simulink model "MotorAsincronoMotorCCCarga"  (Simulink 6.5)
settings: Solver=ode23t  StartTime=0.0  StopTime=4.5  RelTol=1e-6
undefined symbols (not defined in the file): powergui
libraries: powerlib x30, powerlib_extras x3
settings Model: Creator=RS  LastModifiedBy=PC_0
settings SolverCC: SolverResetMethod=Robust

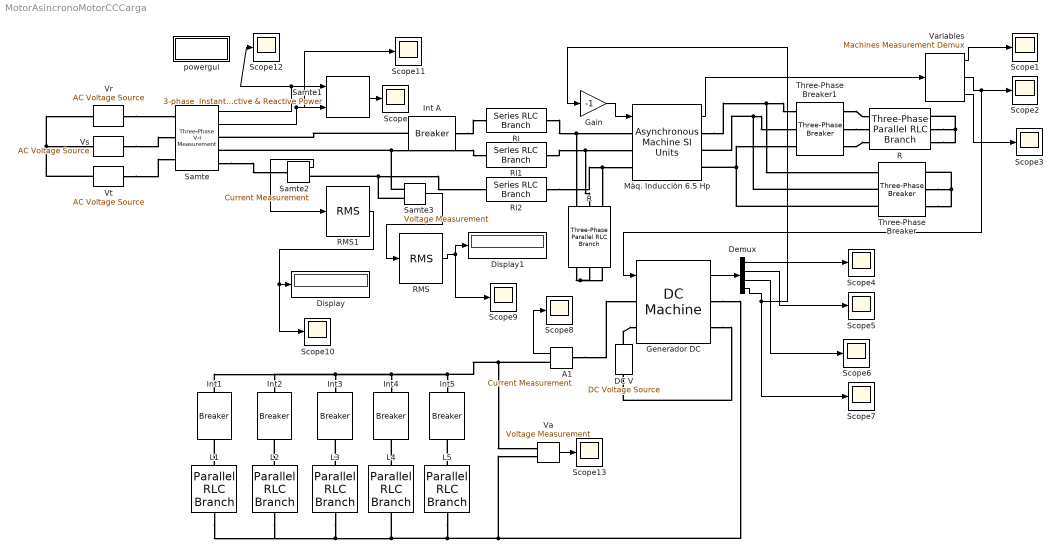
== system MotorAsincronoMotorCCCarga ==
  A1 : powerlib/Measurements/Current Measurement  Orientation=left  DialogController=PMDialogs.PMDefaultMaskDlg  SystemSampleTime=-1  PhasorSimulation=off  OutputType=Complex  PSBequivalent=0
  DC V : powerlib/Electrical Sources/DC Voltage Source  Orientation=up  DialogController=PMDialogs.PMDefaultMaskDlg  SystemSampleTime=-1  Amplitude=190  Measurements=None
  Demux : Demux
  Display : Display
  Display1 : Display
  Gain : Gain  Gain=-1
  Generador DC : powerlib/Machines/DC Machine  DialogController=PMDialogs.PMDefaultMaskDlg  SystemSampleTime=-1  PresetModel=No  MechanicalLoad=Speed w  ShowDetailedParameters=on  RLa="[ 0.5  0.01]"  RLf="[ 240  120]"  Laf=1.8  J=0.05  Bm=0.02  Tf=0  w0=0
  Int A : powerlib/Elements/Breaker  DialogController=PMDialogs.PMDefaultMaskDlg  SystemSampleTime=-1  BreakerResistance=0.01  InitialState=1  SnubberResistance=1e6  SnubberCapacitance=inf  SwitchingTimes=9  External=off  Measurements=None  MoreParameters=off  NoBreakLoop=off
  Int1 : powerlib/Elements/Breaker  Orientation=down  DialogController=PMDialogs.PMDefaultMaskDlg  SystemSampleTime=-1  BreakerResistance=0.01  InitialState=0  SnubberResistance=1e6  SnubberCapacitance=inf  SwitchingTimes=1.5  External=off  Measurements=None  MoreParameters=off  NoBreakLoop=off
  Int2 : powerlib/Elements/Breaker  Orientation=down  DialogController=PMDialogs.PMDefaultMaskDlg  SystemSampleTime=-1  BreakerResistance=0.01  InitialState=0  SnubberResistance=1e6  SnubberCapacitance=inf  SwitchingTimes=1.75  External=off  Measurements=None  MoreParameters=off  NoBreakLoop=off
  Int3 : powerlib/Elements/Breaker  Orientation=down  DialogController=PMDialogs.PMDefaultMaskDlg  SystemSampleTime=-1  BreakerResistance=0.01  InitialState=0  SnubberResistance=1e6  SnubberCapacitance=inf  SwitchingTimes=2  External=off  Measurements=None  MoreParameters=off  NoBreakLoop=off
  Int4 : powerlib/Elements/Breaker  Orientation=down  DialogController=PMDialogs.PMDefaultMaskDlg  SystemSampleTime=-1  BreakerResistance=0.01  InitialState=0  SnubberResistance=1e6  SnubberCapacitance=inf  SwitchingTimes=2.25  External=off  Measurements=None  MoreParameters=off  NoBreakLoop=off
  Int5 : powerlib/Elements/Breaker  Orientation=down  DialogController=PMDialogs.PMDefaultMaskDlg  SystemSampleTime=-1  BreakerResistance=0.01  InitialState=0  SnubberResistance=1e6  SnubberCapacitance=inf  SwitchingTimes=2.5  External=off  Measurements=None  MoreParameters=off  NoBreakLoop=off
  L{1..5} (5 alike) : powerlib/Elements/Parallel RLC Branch  Orientation=down  DialogController=PMDialogs.PMDefaultMaskDlg  PhysicalDomain=powersysdomain  SubClassName=unknown  LeftPortType=p1  RightPortType=p1  LConnTagsString=a  RConnTagsString=__new0  BranchType=R  Resistance=65  Inductance=1e-3  SetiL0=off  InitialCurrent=0  Capacitance=1e-6  Setx0=off  InitialVoltage=0  Measurements=None
  Màq. Inducciòn 6.5 Hp : powerlib/Machines/Asynchronous Machine SI Units  DialogController=PMDialogs.PMDefaultMaskDlg  SystemSampleTime=-1  PresetModel=No  MechanicalLoad=Torque Tm  ShowDetailedParameters=on  RotorType=Wound  ReferenceFrame=Stationary  NominalParameters="[6.5*746    380   50]"  Stator="[0.03   0.00006]"  Rotor="[1.094  0.00496]"  Lm=0.105  Mechanical="[0.041    0.001   2]"  PolePairs=2  InitialConditions="[ 1,0   0,0,0   0,0,0 ]"  Units=1  LoadFlowParameters=0  SimulateSaturation=on  Saturation=[ 0.5 3,6,9,12,15,18,30,50;20,190,380,400,420,440,450,451,452]
  R : powerlib/Elements/Three-Phase Parallel RLC Branch  DialogController=PMDialogs.PMDefaultMaskDlg  PhysicalDomain=powersysdomain  SubClassName=unknown  LeftPortType=p1  RightPortType=p1  LConnTagsString=A|B|C  RConnTagsString=A|B|C  BranchType=R  Resistance=4.2  Inductance=1e-3  Capacitance=1e-6  Measurements=None
  "R " : powerlib/Elements/Three-Phase Parallel RLC Branch  Orientation=down  DialogController=PMDialogs.PMDefaultMaskDlg  PhysicalDomain=powersysdomain  SubClassName=unknown  LeftPortType=p1  RightPortType=p1  LConnTagsString=A|B|C  RConnTagsString=A|B|C  BranchType=R  Resistance=300  Inductance=1e-3  Capacitance=1e-6  Measurements=None
  RMS : powerlib_extras/Measurements/RMS  DialogController=PMDialogs.PMDefaultMaskDlg  SystemSampleTime=-1  f1=50
  RMS1 : powerlib_extras/Measurements/RMS  DialogController=PMDialogs.PMDefaultMaskDlg  SystemSampleTime=-1  f1=50
  Rl : powerlib/Elements/Series RLC Branch  DialogController=PMDialogs.PMDefaultMaskDlg  PhysicalDomain=powersysdomain  SubClassName=unknown  LeftPortType=p1  RightPortType=p1  LConnTagsString=__new0  RConnTagsString=__new0  BranchType=RL  Resistance=0.6  Inductance=0.0049  SetiL0=off  InitialCurrent=0  Capacitance=1e-6  Setx0=off  InitialVoltage=0  Measurements=None
  Rl1 : powerlib/Elements/Series RLC Branch  DialogController=PMDialogs.PMDefaultMaskDlg  PhysicalDomain=powersysdomain  SubClassName=unknown  LeftPortType=p1  RightPortType=p1  LConnTagsString=__new0  RConnTagsString=__new0  BranchType=RL  Resistance=0.6  Inductance=0.0049  SetiL0=off  InitialCurrent=0  Capacitance=1e-6  Setx0=off  InitialVoltage=0  Measurements=None
  Rl2 : powerlib/Elements/Series RLC Branch  DialogController=PMDialogs.PMDefaultMaskDlg  PhysicalDomain=powersysdomain  SubClassName=unknown  LeftPortType=p1  RightPortType=p1  LConnTagsString=__new0  RConnTagsString=__new0  BranchType=RL  Resistance=0.6  Inductance=0.0049  SetiL0=off  InitialCurrent=0  Capacitance=1e-6  Setx0=off  InitialVoltage=0  Measurements=None
  Samte : powerlib/Measurements/Three-Phase V-I Measurement  DialogController=PMDialogs.PMDefaultMaskDlg  SystemSampleTime=-1  VoltageMeasurement=phase-to-phase  SetLabelV=off  LabelV=Vabc  Vpu=off  CurrentMeasurement=yes  SetLabelI=off  LabelI=Iabc  Ipu=off  Pbase=100e6  Vbase=500e3  OutputType=Complex  PhasorSimulation=off  PSBequivalent=0
  Samte1 : powerlib_extras/Measurements/3-phase  Instantaneous  Active & Reactive Power  DialogController=PMDialogs.PMDefaultMaskDlg  SystemSampleTime=-1
  Samte2 : powerlib/Measurements/Current Measurement  DialogController=PMDialogs.PMDefaultMaskDlg  SystemSampleTime=-1  PhasorSimulation=off  OutputType=Complex  PSBequivalent=0
  Samte3 : powerlib/Measurements/Voltage Measurement  DialogController=PMDialogs.PMDefaultMaskDlg  SystemSampleTime=-1  PhasorSimulation=off  OutputType=Complex  PSBequivalent=0
  Scope{,1..13} (14 alike) : Scope
      Scope settings: MaxDataPoints=10000000  SampleInput=on  SampleTime=10e-6
      Scope1 settings: MaxDataPoints=10000000  SampleInput=on  SampleTime=10e-6
      Scope10 settings: SaveName=ScopeData10  MaxDataPoints=10000000  SampleInput=on  SampleTime=10e-6
      Scope11 settings: SaveName=ScopeData11  MaxDataPoints=10000000  SampleInput=on  SampleTime=10e-6
      Scope12 settings: SaveName=ScopeData12  MaxDataPoints=10000000  SampleInput=on  SampleTime=10e-6
      Scope13 settings: SaveName=ScopeData13  MaxDataPoints=10000000  SampleInput=on  SampleTime=10e-6
      Scope2 settings: SaveName=ScopeData2  MaxDataPoints=10000000  SampleInput=on  SampleTime=10e-6
      Scope3 settings: SaveName=ScopeData3  MaxDataPoints=10000000  SampleInput=on  SampleTime=10e-6
      Scope4 settings: SaveName=ScopeData4  MaxDataPoints=10000000  SampleInput=on  SampleTime=10e-6
      Scope5 settings: SaveName=ScopeData5  MaxDataPoints=10000000  SampleInput=on  SampleTime=10e-6
      Scope6 settings: SaveName=ScopeData6  MaxDataPoints=10000000  SampleInput=on  SampleTime=10e-6
      Scope7 settings: SaveName=ScopeData7  MaxDataPoints=10000000  SampleInput=on  SampleTime=10e-6
      Scope8 settings: SaveName=ScopeData8  MaxDataPoints=10000000  SampleInput=on  SampleTime=10e-6
      Scope9 settings: SaveName=ScopeData9  MaxDataPoints=10000000  SampleInput=on  SampleTime=10e-6
  Three-Phase Breaker : powerlib/Elements/Three-Phase Breaker  DialogController=PMDialogs.PMDefaultMaskDlg  SystemSampleTime=-1  InitialState=open  SwitchA=on  SwitchB=on  SwitchC=on  SwitchTimes=1  External=off  BreakerResistance=0.001  SnubberResistance=1e6  SnubberCapacitance=inf  Measurements=None
  Three-Phase Breaker1 : powerlib/Elements/Three-Phase Breaker  DialogController=PMDialogs.PMDefaultMaskDlg  SystemSampleTime=-1  InitialState=closed  SwitchA=on  SwitchB=on  SwitchC=on  SwitchTimes=1  External=off  BreakerResistance=0.001  SnubberResistance=1e6  SnubberCapacitance=inf  Measurements=None
  Va : powerlib/Measurements/Voltage Measurement  DialogController=PMDialogs.PMDefaultMaskDlg  SystemSampleTime=-1  PhasorSimulation=off  OutputType=Complex  PSBequivalent=0
  Variables : powerlib/Machines/Machines Measurement Demux  DialogController=PMDialogs.PMDefaultMaskDlg  SystemSampleTime=-1  machType=Asynchronous  ssm1=on  ssm2=on  ssm3=on  ssm4=on  ssm5=on  ssm6=on  sm1=off  sm2=off  sm3=off  sm4=off  sm5=off  sm6=off  sm7=off  sm8=on  sm9=off  sm10=off  sm11=off  sm115=off  sm12=off  sm13=off  sm14=off  asm1=off  asm2=off  asm3=off  asm4=off  asm5=on  asm6=off  asm7=off  asm8=off  asm9=on  asm10=on  asm11=off  pmsm1=on  pmsm2=on  pmsm3=on  pmsm4=off  pmsm5=on  pmsm6=on  pmsm7=on  lastType=1
  Vr : powerlib/Electrical Sources/AC Voltage Source  DialogController=PMDialogs.PMDefaultMaskDlg  SystemSampleTime=-1  Amplitude=218.8*sqrt(2)  Phase=0  Frequency=50  SampleTime=0  Measurements=None
  Vs : powerlib/Electrical Sources/AC Voltage Source  DialogController=PMDialogs.PMDefaultMaskDlg  SystemSampleTime=-1  Amplitude=216.7*sqrt(2)  Phase=-118.1  Frequency=50  SampleTime=0  Measurements=None
  Vt : powerlib/Electrical Sources/AC Voltage Source  DialogController=PMDialogs.PMDefaultMaskDlg  SystemSampleTime=-1  Amplitude=214.9*sqrt(2)  Phase=119.7  Frequency=50  SampleTime=0  Measurements=None
  powergui : Subsystem  AncestorBlock=powerlib/powergui  InitFcn=powergui( 'InitFcn_Callback' , gcb , 0 , [ ] );  mask(PSB option menu block){SimulationMode=Continuous, SampleTime=50e-6, echomessages=off, RestoreLinks=warning, x0status=blocks, Frange=[0:2:500], Ylog=off, Xlog=on, ShowGrid=off, save=off, variable=ZData, structure=ScopeData1, ZoomFFT=off, StartTime=4, cycles=10, DisplayStyle=2, fundamental=50, FreqAxis=off, MaxFrequency=1000, frequencyindice=50, frequencyindicesteady=1, RmsSteady=1, display=off, Ts=0, frequency=60, methode=off, HookPort=off, Interpol=off}
      mask prompts: SimulationMode "Simulation mode"; SampleTime "Sample time Ts (when simulation mode is Discrete) (s)"; echomessages "Echo  Messages"; RestoreLinks "Restore disabled links"; x0status "Initial electrical states status"; Frange "Impedance tool: Frequency Range"; Ylog "Impedance tool: Log impedance"; Xlog "Impedance tool: log Frequency"; ShowGrid "Impedance tool: grid"; save "Impedance tool: Save Data To Workspace"; variable "Impedance tool: Variable Name"; structure "Structure Name (PSBFFTSCOPE)"; ZoomFFT "ZoomFFT (PSBFFTSCOPE)"; StartTime "Start Time (PSBFFTSCOPE)"; cycles "Cycles (PSBFFTSCOPE)"; DisplayStyle "Display style (PSBFFTSCOPE)"; fundamental "Fundamental (PSBFFTSCOPE)"; FreqAxis "Frequency Axis (PSBFFTSCOPE)"; MaxFrequency "Max Frequency (PSBFFTSCOPE)"; frequencyindice "Load flow frequency (Hz)"; frequencyindicesteady "Frequency indice (STEADYSTATE)"; RmsSteady "RMS display (STEADYSTATE)"; display "Display Results"; Ts "OBSOLETE 1"; frequency "Phasor frequency (Hz)"; methode "Phasor simulation"; HookPort "Hook port"; Interpol "Interpolate"
      mask init:
      | powerlibroot = which('powersysdomain');
      | PSBroot = powerlibroot(1:end-16);
      | %
      | switch SimulationMode
      | 	case 1
      | 		message=sprintf('Continuous');
      | 	case 2
      |         SampleTimeeval=evalin('base',SampleTime,'NaN');
      |         if isnan(SampleTimeeval)
      |             message=sprintf('Warning !!,\nUndefined sample time');
      |         else
      |             message=sprintf('Discrete,\nTs = %.4g s.',SampleTimeeval);
      |         end
      | 	case 3
      | 		message=sprintf('Phasors');
      | end
      | if strcmp(bdroot,'powerlib')
      |   message='powergui';
      | end
      | power_initmask();
      settings: CopyFcn=powergui( 'Copy_Callback' , gcb , 0 , [ ] );  ModelCloseFcn=powergui( 'CloseButton_Callback' , gcb , [ ] , [ ] );  PreSaveFcn=powergui( 'CloseButton_Callback' , gcb , [ ] , [ ] );  NameChangeFcn=powergui( 'NameChangeFcn_Callback' , gcb , 0 , [ ] );
      settings: DeleteFcn=|
      | powergui( 'Copy_Callback' , gcb , 1 , [ ] );
      | powergui( 'CloseButton_Callback' , gcb , [ ] , [ ] );
      settings: OpenFcn=|
      | if (power_openblockproxy ('secondary'))
      | powergui(gcb,'PM')
      | end;
      mask Help: web(psbhelp)
      mask StyleString: popup(Continuous|Discrete|Phasor),edit,checkbox,popup(yes|warning|no),popup(blocks|steady|zero),edit,checkbox,checkbox,checkbox,checkbox,edit,edit,checkbox,edit,edit,edit,edit,checkbox,edit,edit,edit,edit,checkbox,edit,edit,checkbox,checkbox,checkbox
      mask CallbackString: ||||||||||||||||||||||||||powergui('HookPort',[],[],gcb);|
      mask Display: disp(message)
  wires:
  Samte/1 -> Samte1/1, Scope12/1
  Samte/2 -> Samte1/2, Scope11/1
  Samte1/1 -> Scope/1
  Màq. Inducciòn 6.5 Hp/1 -> Variables/1
  Generador DC/1 -> Demux/1
  Gain/1 -> Màq. Inducciòn 6.5 Hp/1
  Demux/4 -> Gain/1, Scope7/1
  Demux/1 -> Scope4/1
  Demux/2 -> Scope5/1
  Demux/3 -> Scope6/1
  Va/1 -> Scope13/1
  RMS1/1 -> Display/1, Scope10/1
  Variables/3 -> Scope3/1
  Samte2/1 -> RMS1/1
  Samte3/1 -> RMS/1
  RMS/1 -> Display1/1, Scope9/1
  Variables/1 -> Scope1/1
  Variables/2 -> Generador DC/1, Scope2/1
  A1/1 -> Scope8/1
  connections:
  Samte3/LConn1 -- Samte/RConn2 -- Rl1/LConn1
  Samte3/LConn2 -- Samte2/RConn1 -- Rl2/LConn1
  DC V/RConn1 -- Generador DC/LConn2
  L1/LConn1 -- Int1/RConn1
  L2/LConn1 -- Int2/RConn1
  L3/LConn1 -- Int3/RConn1
  L4/LConn1 -- Int4/RConn1
  L5/LConn1 -- Int5/RConn1
  Generador DC/RConn1 -- L5/RConn1 -- L1/RConn1 -- L2/RConn1 -- L3/RConn1 -- L4/RConn1 -- Va/LConn2
  "R "/RConn1 -- "R "/RConn3 -- "R "/RConn2
  A1/LConn1 -- Generador DC/LConn1
  Vt/LConn1 -- Vr/LConn1 -- Vs/LConn1
  Vr/RConn1 -- Samte/LConn1
  Vs/RConn1 -- Samte/LConn2
  Vt/RConn1 -- Samte/LConn3
  Samte/RConn3 -- Samte2/LConn1
  Int A/RConn1 -- Rl/LConn1
  Rl/RConn1 -- Màq. Inducciòn 6.5 Hp/LConn1 -- "R "/LConn1
  Rl1/RConn1 -- Màq. Inducciòn 6.5 Hp/LConn2 -- "R "/LConn2
  Rl2/RConn1 -- Màq. Inducciòn 6.5 Hp/LConn3 -- "R "/LConn3
  Màq. Inducciòn 6.5 Hp/RConn1 -- Three-Phase Breaker/LConn1 -- Three-Phase Breaker1/LConn1
  Three-Phase Breaker/LConn2 -- Màq. Inducciòn 6.5 Hp/RConn2 -- Three-Phase Breaker1/LConn2
  Three-Phase Breaker/LConn3 -- Màq. Inducciòn 6.5 Hp/RConn3 -- Three-Phase Breaker1/LConn3
  Three-Phase Breaker1/RConn1 -- R/LConn1
  Three-Phase Breaker1/RConn2 -- R/LConn2
  Three-Phase Breaker1/RConn3 -- R/LConn3
  Three-Phase Breaker/RConn3 -- Three-Phase Breaker/RConn1 -- Three-Phase Breaker/RConn2
  R/RConn3 -- R/RConn1 -- R/RConn2
  A1/RConn1 -- Int1/LConn1 -- Int2/LConn1 -- Int3/LConn1 -- Int4/LConn1 -- Int5/LConn1 -- Va/LConn1
  Generador DC/RConn2 -- DC V/LConn1
  Int A/LConn1 -- Samte/RConn1

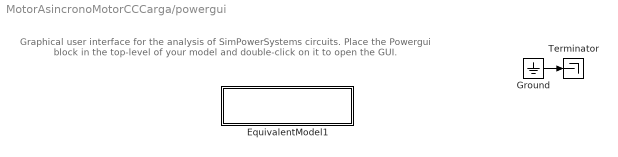
== system MotorAsincronoMotorCCCarga/powergui ==
  note: Graphical user interface for the analysis of  SimPowerSystems circuits.
      | Place the Powergui block in the top-level of your model and double-click
      | on it to open the GUI.
  EquivalentModel1 : Subsystem
      mask init:
      | SPS = get_param(gcbh,'UserData');
      | if isempty(SPS)
      |     A=0;
      |     B=0;
      |     C=0;
      |     D=0;
      |     x0=0;
      |     SwitchResistance=1;
      |     SwitchType=1;
      |     SwitchGateInitialValue=1;
      |     OutputsToResetToZero=1;
      | else
      | 	A=SPS.A;
      |     B=SPS.B;
      |     C=SPS.C;
      |     D=SPS.D;
      |     x0=SPS.x0;
      |     SwitchResistance=SPS.SwitchResistance;
      |     SwitchType=SPS.SwitchType;
      |     SwitchGateInitialValue=SPS.SwitchGateInitialValue;
      |     OutputsToResetToZero=SPS.YSwitchCurrent;
      | end
      mask Display:
      | color('blue')
      | disp('EQUIVALENT CIRCUIT')
  Ground : Ground
  Terminator : Terminator
  wires:
  Ground/1 -> Terminator/1

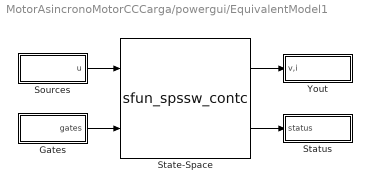
== system MotorAsincronoMotorCCCarga/powergui/EquivalentModel1 ==
  Gates : Subsystem
  Sources : Subsystem
  State-Space : S-Function  FunctionName=sfun_spssw_contc  Parameters=A, B, C, D, x0, SwitchResistance ,SwitchType, SwitchGateInitialValue, OutputsToResetToZero
  Status : Subsystem
  Yout : Subsystem
  wires:
  Gates/1(gates) -> State-Space/2
  Sources/1(u) -> State-Space/1
  State-Space/2 -> Status/1(status)
  State-Space/1 -> Yout/1(v,i)

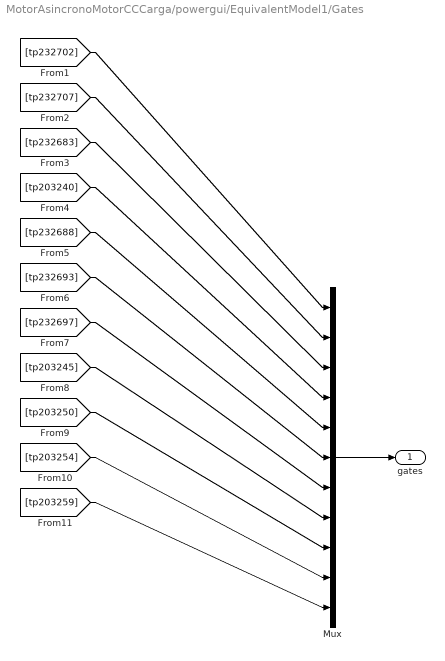
== system MotorAsincronoMotorCCCarga/powergui/EquivalentModel1/Gates ==
  Mux : Mux  Inputs=[1 1 1 1 1 1 1 1 1 1 1]
  gates : Outport
  wires:
  Mux/1 -> gates/1
  [tp232702] -> Mux/1
  [tp232707] -> Mux/2
  [tp232683] -> Mux/3
  [tp203240] -> Mux/4
  [tp232688] -> Mux/5
  [tp232693] -> Mux/6
  [tp232697] -> Mux/7
  [tp203245] -> Mux/8
  [tp203250] -> Mux/9
  [tp203254] -> Mux/10
  [tp203259] -> Mux/11

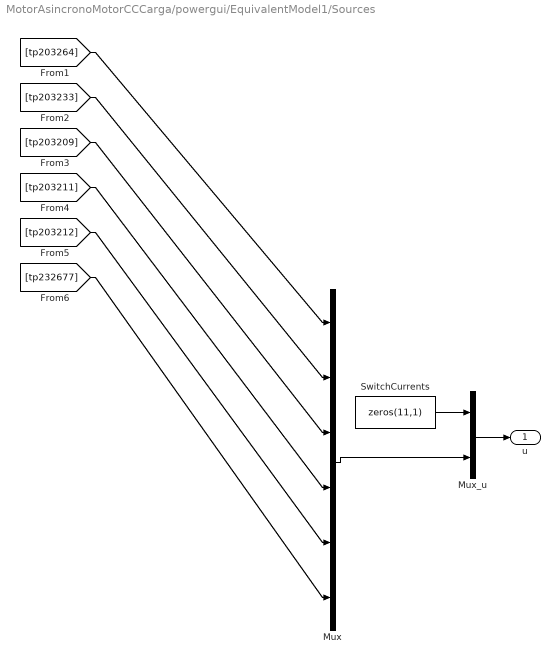
== system MotorAsincronoMotorCCCarga/powergui/EquivalentModel1/Sources ==
  Mux : Mux  Inputs=[4 1 1 1 1 1]
  Mux_u : Mux  Inputs=[11 9]
  SwitchCurrents : Constant  Value=zeros(11,1)  OutDataType=sfix(16)  ConRadixGroup=Use specified scaling  OutScaling=2^0  SampleTime=inf  FramePeriod=inf
  u : Outport
  wires:
  Mux/1 -> Mux_u/2
  SwitchCurrents/1 -> Mux_u/1
  Mux_u/1 -> u/1
  [tp203264] -> Mux/1
  [tp203233] -> Mux/2
  [tp203209] -> Mux/3
  [tp203211] -> Mux/4
  [tp203212] -> Mux/5
  [tp232677] -> Mux/6

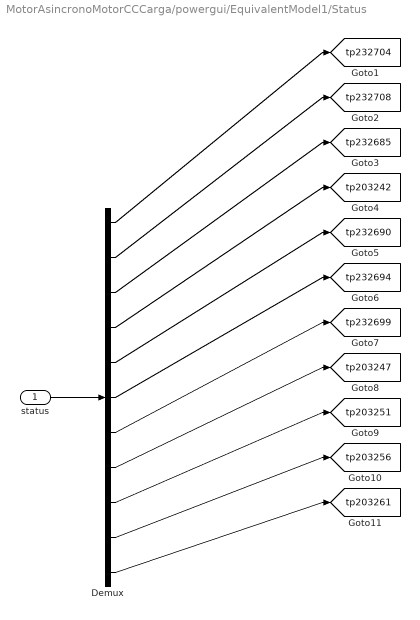
== system MotorAsincronoMotorCCCarga/powergui/EquivalentModel1/Status ==
  status : Inport
  Demux : Demux  Outputs=[1 1 1 1 1 1 1 1 1 1 1]
  tag scope: tp203242=global, tp203247=global, tp203251=global, tp203256=global, tp203261=global, tp232685=global, tp232690=global, tp232694=global, tp232699=global, tp232704=global, tp232708=global
  wires:
  status/1 -> Demux/1
  Demux/1 -> [tp232704]
  Demux/2 -> [tp232708]
  Demux/3 -> [tp232685]
  Demux/4 -> [tp203242]
  Demux/5 -> [tp232690]
  Demux/6 -> [tp232694]
  Demux/7 -> [tp232699]
  Demux/8 -> [tp203247]
  Demux/9 -> [tp203251]
  Demux/10 -> [tp203256]
  Demux/11 -> [tp203261]

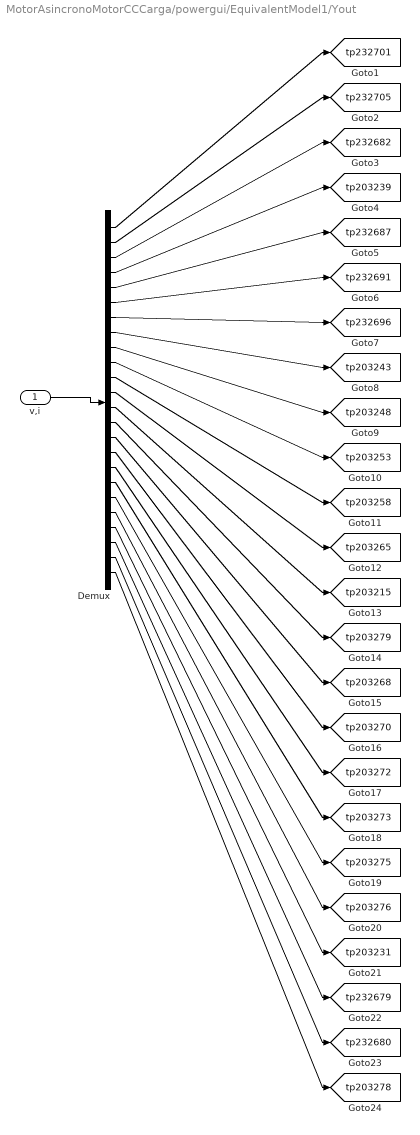
== system MotorAsincronoMotorCCCarga/powergui/EquivalentModel1/Yout ==
  v,i : Inport
  Demux : Demux  Outputs=[1 1 1 1 1 1 1 1 1 1 1 4 1 1 1 1 1 1 1 1 1 1 1 1]
  tag scope: tp203215=global, tp203231=global, tp203239=global, tp203243=global, tp203248=global, tp203253=global, tp203258=global, tp203265=global, tp203268=global, tp203270=global, tp203272=global, tp203273=global, tp203275=global, tp203276=global, tp203278=global, tp203279=global, tp232679=global, tp232680=global, tp232682=global, tp232687=global, tp232691=global, tp232696=global, tp232701=global, tp232705=global
  wires:
  v,i/1 -> Demux/1
  Demux/1 -> [tp232701]
  Demux/2 -> [tp232705]
  Demux/3 -> [tp232682]
  Demux/4 -> [tp203239]
  Demux/5 -> [tp232687]
  Demux/6 -> [tp232691]
  Demux/7 -> [tp232696]
  Demux/8 -> [tp203243]
  Demux/9 -> [tp203248]
  Demux/10 -> [tp203253]
  Demux/11 -> [tp203258]
  Demux/12 -> [tp203265]
  Demux/13 -> [tp203215]
  Demux/14 -> [tp203279]
  Demux/15 -> [tp203268]
  Demux/16 -> [tp203270]
  Demux/17 -> [tp203272]
  Demux/18 -> [tp203273]
  Demux/19 -> [tp203275]
  Demux/20 -> [tp203276]
  Demux/21 -> [tp203231]
  Demux/22 -> [tp232679]
  Demux/23 -> [tp232680]
  Demux/24 -> [tp203278]
